simulink model "store_and_retrieve_input"  (R2020a)
settings: Solver=FixedStepDiscrete  StartTime=0.0  StopTime=840000  RelTol=1e-3
libraries: hdlsllib x2, simulink x1
settings Model: FPTRunName=FPA_Reference  PacingRate=40  Creator=BuccelliLab  LastModifiedBy=diflo
settings SolverCC: AutoInsertRateTranBlk=on  MinimalZcImpactIntegration=on
settings DataIOCC: LimitDataPoints=on  SaveOutput=off  SaveTime=off  ReturnWorkspaceOutputs=off
settings OptimizationCC: BlockReduction=off  ConditionallyExecuteInputs=off  DefaultParameterBehavior=Inlined  LifeSpan=inf
settings DebuggingCC: SignalRangeChecking=warning  ReadBeforeWriteMsg=DisableAll  WriteAfterWriteMsg=DisableAll  WriteAfterReadMsg=DisableAll  AlgebraicLoopMsg=error  MultiTaskDSMMsg=none  SingleTaskRateTransMsg=error  ParameterDowncastMsg=warning  ParameterOverflowMsg=warning  AllowSymbolicDim=off  StrictBusMsg=ErrorOnBusTreatedAsVector  SFUnexpectedBacktrackingDiag=warning  SFNoUnconditionalDefaultTransitionDiag=warning  SFExecutionAtInitializationDiag=none  ArithmeticOperatorsInVariantConditions=warning
settings HardwareCC: ProdBitPerPointer=32  ProdBitPerSizeT=32  ProdBitPerPtrDiffT=32  ProdLargestAtomicFloat=None  ProdIntDivRoundTo=Undefined  ProdEndianess=Unspecified  ProdWordSize=32  ProdHWDeviceType=ASIC/FPGA->ASIC/FPGA  TargetBitPerPointer=64  TargetBitPerSizeT=64  TargetBitPerPtrDiffT=64  TargetLongLongMode=on  TargetIntDivRoundTo=Zero  TargetEndianess=LittleEndian  TargetWordSize=64  TargetHWDeviceType=Custom Processor->MATLAB Host Computer  ProdEqTarget=off
settings ModelReferenceCC: UpdateModelReferenceTargets=IfOutOfDate
settings SFSimCC: SFSimEcho=off  SimUseLocalCustomCode=off  CustomCodeUndefinedFunction=UseInterfaceOnly
settings RTWCC: RTWUseLocalCustomCode=off
settings CodeAppCC: StateflowObjectComments=on
settings GRTTargetCC: TargetLangStandard=C89/C90 (ANSI)
settings ConfigComp: CovScope=ReferencedModels  CovMetricSettings=dw  CovHtmlReporting=on  CovSaveCumulativeToWorkspaceVar=on  CovSaveSingleToWorkspaceVar=on  CovExternalEMLEnable=off  CovSFcnEnable=off

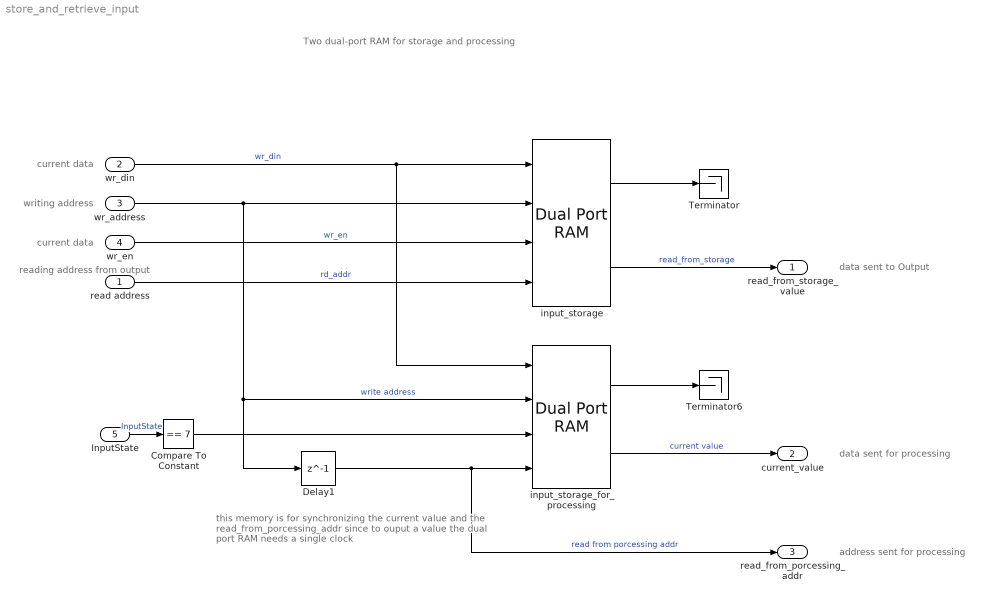
== system store_and_retrieve_input ==
  note: Two dual-port RAM for storage and processing
  note: current data
  note: data sent to Output
  note: data sent for processing
  note: this memory is for synchronizing the current value and
      | the read_from_porcessing_addr since to ouput a value
      | the dual port RAM needs a single clock
  note: current data
  note: reading address
      | from output
  note: address sent for processing
  note: writing address
  read address : Inport  OutDataTypeStr=fixdt(0,9,0)  PortDimensions=1  SampleTime=[1,0]
  wr_din : Inport  Port=2  OutDataTypeStr=uint16  PortDimensions=1  SampleTime=[1,0]
  wr_address : Inport  Port=3  OutDataTypeStr=fixdt(0,9,0)  PortDimensions=1  SampleTime=[1,0]
  wr_en : Inport  Port=4  OutDataTypeStr=boolean  PortDimensions=1  SampleTime=[1,0]
  InputState : Inport  Port=5  OutDataTypeStr=uint8  PortDimensions=1  SampleTime=[1,0]
  Compare To Constant : simulink/Logic and Bit Operations/Compare To Constant  relop===  const=7  OutDataTypeStr=boolean
  Delay1 : Delay  DelayLength=1  InitialCondition=0
  Terminator : Terminator
  Terminator6 : Terminator
  input_storage : hdlsllib/HDL RAMs/Dual Port RAM  ram_size=9
      settings: SourceProductBaseCode=SL
  input_storage_for_processing : hdlsllib/HDL RAMs/Dual Port RAM  ram_size=9
      settings: SourceProductBaseCode=SL
  read_from_storage_value : Outport  OutDataTypeStr=uint16  PortDimensions=1  SampleTime=[1,0]
  current_value : Outport  Port=2  OutDataTypeStr=uint16  PortDimensions=1  SampleTime=[1,0]
  read_from_porcessing_addr : Outport  Port=3  OutDataTypeStr=fixdt(0,9,0)  PortDimensions=1  SampleTime=[1,0]
  wires:
  wr_en/1 -> input_storage/3  "wr_en"
  InputState/1 -> Compare To Constant/1  "InputState"
  Compare To Constant/1 -> input_storage_for_processing/3
  input_storage_for_processing/2 -> current_value/1  "current value"
  Delay1/1 -> input_storage_for_processing/4, read_from_porcessing_addr/1  "read from porcessing addr"
  input_storage/1 -> Terminator/1
  wr_address/1 -> input_storage/2, input_storage_for_processing/2, Delay1/1  "write address"
  wr_din/1 -> input_storage/1, input_storage_for_processing/1  "wr_din"
  input_storage/2 -> read_from_storage_value/1  "read_from_storage"
  input_storage_for_processing/1 -> Terminator6/1
  read address/1 -> input_storage/4  "rd_addr"
